simulink model "course_hold_AP_2e"  (R2015a)
settings: Solver=ode45  SolverMode=SingleTasking  StartTime=0.0  StopTime=300  RelTol=1e-3
values from neighbouring files (symbols this model uses):
  g = 9.81    [constants.m]    (also in prob_2_e.m; rlocus.m = -h)
  kd_fi = (2*zeta_fi*omega_fi-alpha_fi1)/alpha_fi2    [constants.m]    (also in prob_2_e.m)
  ki_chi = omega_chi^2*V_g/g    [constants.m]    (also in prob_2_e.m)
  ki_fi = -0    (= 0)    [constants.m]    (also in prob_2_e.m)
  kp_chi = 2*zeta_chi*omega_chi*V_g/g    [constants.m]    (also in prob_2_e.m)
  kp_fi = -2    [constants.m]    (also in prob_2_e.m)
  V_g = 580/3.6    (= 161.111111111)    [constants.m]    (also in prob_2_e.m)
libraries: simulink_extras x2
settings Model: CovMetricSettings=dwe  CovHtmlReporting=off  covSaveCumulativeToWorkspaceVar=off  CovSaveSingleToWorkspaceVar=off  CovExternalEMLEnable=on  Creator=marti  LastModifiedBy=Anders Vagle
settings DataIOCC: LimitDataPoints=off  SaveFormat=Dataset
settings DebuggingCC: SFUnexpectedBacktrackingDiag=error  SFNoUnconditionalDefaultTransitionDiag=error
settings HardwareCC: ProdBitPerPointer=64  ProdLargestAtomicFloat=Float  ProdIntDivRoundTo=Zero  ProdEndianess=LittleEndian  ProdHWDeviceType=Specified
settings ModelReferenceCC: PropagateSignalLabelsOutOfModel=on
settings GRTTargetCC: TargetLangStandard=C99 (ISO)  GeneratePreprocessorConditionals=Use local settings

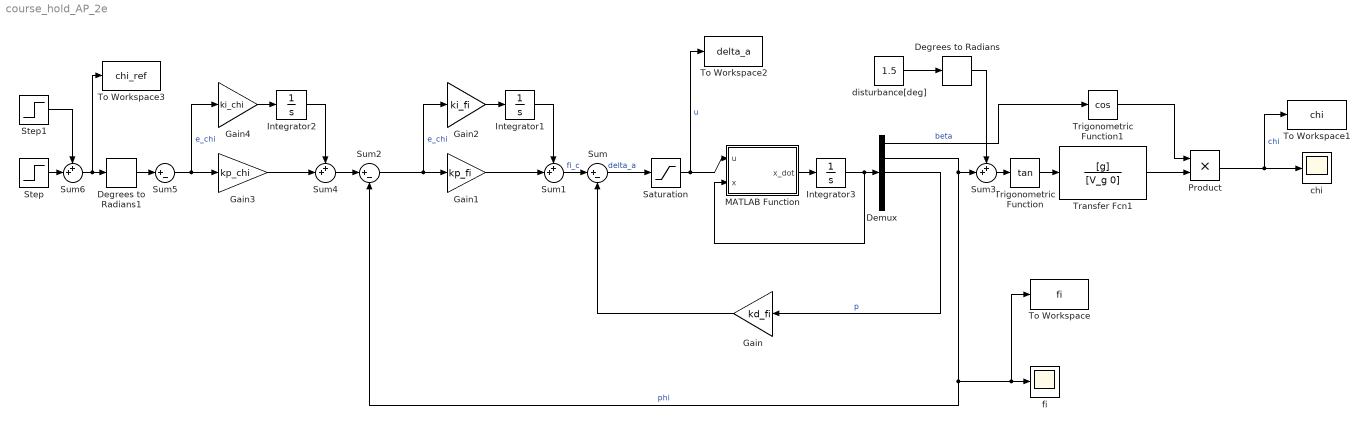
== system course_hold_AP_2e ==
  Degrees to Radians : simulink_extras/Transformations/Degrees to Radians
  Degrees to Radians1 : simulink_extras/Transformations/Degrees to Radians
  Demux : Demux  Outputs=5
  Gain : Gain  Gain=kd_fi
  Gain1 : Gain  Gain=kp_fi
  Gain2 : Gain  Gain=ki_fi
  Gain3 : Gain  Gain=kp_chi
  Gain4 : Gain  Gain=ki_chi
  Integrator1 : Integrator
  Integrator2 : Integrator
  Integrator3 : Integrator
  MATLAB Function : MATLAB Function  TreatAsAtomicUnit=on
  Product : Product
  Saturation : Saturate  UpperLimit=30/180*pi  LowerLimit=-30/180*pi
  Step : Step  Time=50  After=15  SampleTime=0
  Step1 : Step  Time=150  After=-15  SampleTime=0
  Sum : Sum  Inputs=|+-
  Sum{1,3..4,6} (4 alike) : Sum  Inputs=++|
  Sum2 : Sum  Inputs=|+-
  Sum5 : Sum  Inputs=|+-
  To Workspace : ToWorkspace  VariableName=fi  SaveFormat=Timeseries  SampleTime=-1
  To Workspace1 : ToWorkspace  VariableName=chi  SaveFormat=Timeseries  SampleTime=-1
  To Workspace2 : ToWorkspace  VariableName=delta_a  SaveFormat=Timeseries  SampleTime=-1
  To Workspace3 : ToWorkspace  VariableName=chi_ref  SaveFormat=Timeseries  SampleTime=-1
  Transfer Fcn1 : TransferFcn  Numerator=[g]  Denominator=[V_g 0]
  Trigonometric Function : Trigonometry  Operator=tan
  Trigonometric Function1 : Trigonometry  Operator=cos
  chi : Scope
      settings: YMin=-10  YMax=10
  disturbance[deg] : Constant  Value=1.5
  fi : Scope
      settings: YMin=-10  YMax=10
  wires:
  Gain/1 -> Sum/2
  Gain2/1 -> Integrator1/1
  Sum1/1 -> Sum/1  "fi_c"
  Integrator1/1 -> Sum1/1
  Gain1/1 -> Sum1/2
  Sum2/1 -> Gain2/1, Gain1/1  "e_chi"
  Demux/2 -> To Workspace/1, fi/1, Sum2/2, Sum3/2  "phi"
  Gain4/1 -> Integrator2/1
  Integrator2/1 -> Sum4/1
  Gain3/1 -> Sum4/2
  Sum5/1 -> Gain4/1, Gain3/1  "e_chi"
  Sum/1 -> Saturation/1  "delta_a"
  Sum4/1 -> Sum2/1
  Degrees to Radians1/1 -> Sum5/1
  disturbance[deg]/1 -> Degrees to Radians/1
  Degrees to Radians/1 -> Sum3/1
  Step/1 -> Sum6/2
  Sum6/1 -> To Workspace3/1, Degrees to Radians1/1
  Step1/1 -> Sum6/1
  Sum3/1 -> Trigonometric Function/1
  Trigonometric Function/1 -> Transfer Fcn1/1
  Demux/1 -> Trigonometric Function1/1  "beta"
  Transfer Fcn1/1 -> Product/2
  Trigonometric Function1/1 -> Product/1
  Product/1 -> To Workspace1/1, chi/1  "chi"
  Saturation/1 -> MATLAB Function/1(u), To Workspace2/1  "u"
  MATLAB Function/1(x_dot) -> Integrator3/1
  Integrator3/1 -> MATLAB Function/2(x), Demux/1
  Demux/3 -> Gain/1  "p"

== matlab function course_hold_AP_2e/MATLAB Function ==
  data: u input; x_dot output; x input
function x_dot = fcn(u, x)
% State-space matrices
A = [-0.322, 0.052, 0.028, -1.12, 0.002;
     0, 0, 1, -0.001, 0;
     -10.6, 0, -2.87, 0.46, -0.65;
     6.87, 0, -0.04, -0.32, -0.02;
     0, 0, 0, 0, -7.5];

B = [0; 0; 0; 0; 7.5;];
        
x_dot = A*x+B*u;
